simulink model "triggered"  (R2024b)
settings: Solver=VariableStepAuto  StartTime=0.0  StopTime=10.0  RelTol=1e-3  EnableMultiTasking=on
settings Model: Creator=nicholas  LastModifiedBy=trishkaya.harisunker
settings SolverCC: AlgebraicLoopSolver=TrustRegion
settings DataIOCC: LimitDataPoints=on  SignalLoggingName=sigsOut
settings OptimizationCC: ReuseModelBlockBuffer=off  ExpressionDepthLimit=2147483647  InitFltsAndDblsToZero=on  LifeSpan=inf
settings DebuggingCC: CheckExecutionContextPreStartOutputMsg=on  UnconnectedInputMsg=warning  UnconnectedOutputMsg=warning  UnconnectedLineMsg=warning  PregeneratedLibrarySubsystemCodeDiagnostic=none  SubsystemReferenceDiagnosticForUnitTest=warning
settings HardwareCC: ProdBitPerPointer=32  ProdBitPerSizeT=32  ProdBitPerPtrDiffT=32  ProdLargestAtomicFloat=None  ProdIntDivRoundTo=Undefined  ProdEndianess=Unspecified  ProdWordSize=32  ProdHWDeviceType=32-bit Generic  TargetUnknown=on
settings ModelReferenceCC: EnableRefExpFcnMdlSchedulingChecks=on  PropagateSignalLabelsOutOfModel=off
settings SFSimCC: SimUseLocalCustomCode=off
settings RTWCC: RTWUseLocalCustomCode=off  GPUComputeCapability=3.5  DLArmComputeVersion=19.05
settings CodeAppCC: StateflowObjectComments=on
settings GRTTargetCC: TargetFcnLib=ansi_tfl_tmw.mat  TargetLangStandard=C89/C90 (ANSI)  CombineOutputUpdateFcns=off  GRTInterface=on
settings ConfigComp: CovMetricSettings=dw  CovSaveCumulativeToWorkspaceVar=on  CovSaveSingleToWorkspaceVar=on  CovExternalEMLEnable=off  CovSFcnEnable=off

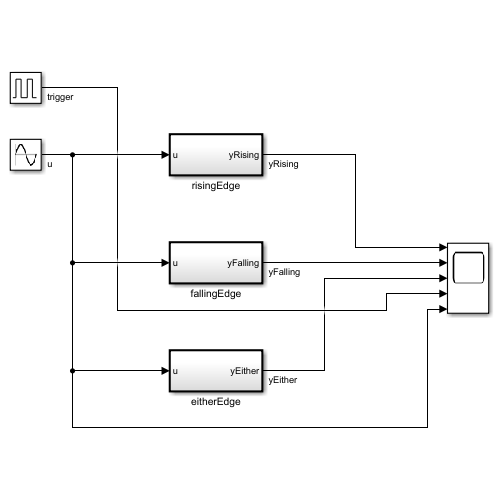
[thumbnail: Simulink's stored preview of the top-level diagram]
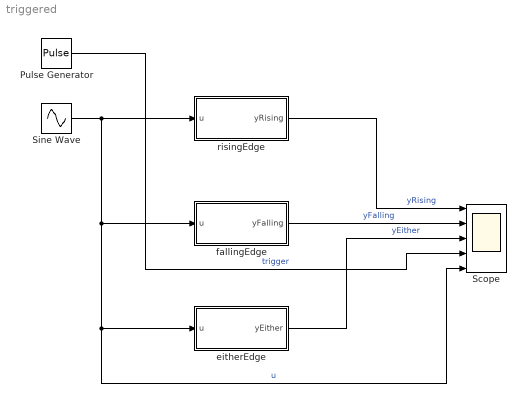
== system triggered ==
  Pulse Generator : DiscretePulseGenerator  PulseType=Time based  Amplitude=4  PulseWidth=50
  Scope : Scope  NumInputPorts=5
  Sine Wave : Sin  Amplitude=4  SampleTime=0
  eitherEdge : Subsystem  TreatAsAtomicUnit=on
  fallingEdge : Subsystem  TreatAsAtomicUnit=on
  risingEdge : Subsystem  TreatAsAtomicUnit=on
  wires:
  fallingEdge/1(yFalling) -> Scope/2  "yFalling"
  risingEdge/1(yRising) -> Scope/1  "yRising"
  eitherEdge/1(yEither) -> Scope/3  "yEither"
  Sine Wave/1 -> risingEdge/1(u), fallingEdge/1(u), Scope/5, eitherEdge/1(u)  "u"
  Pulse Generator/1 -> Scope/4  "trigger"

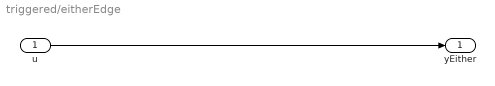
== system triggered/eitherEdge ==
  u : Inport
  yEither : Outport  VectorParamsAs1DForOutWhenUnconnected=off
  wires:
  u/1 -> yEither/1

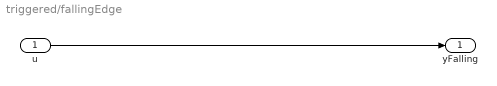
== system triggered/fallingEdge ==
  u : Inport
  yFalling : Outport  VectorParamsAs1DForOutWhenUnconnected=off
  wires:
  u/1 -> yFalling/1

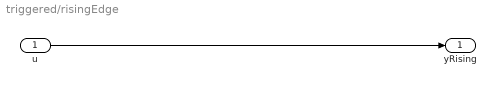
== system triggered/risingEdge ==
  u : Inport
  yRising : Outport  VectorParamsAs1DForOutWhenUnconnected=off
  wires:
  u/1 -> yRising/1
